simulink model "ex6"  (R2021a)
settings: Solver=VariableStepAuto  StartTime=0.0  StopTime=20  RelTol=1e-8
values from neighbouring files (symbols this model uses):
  gamma = 10    [aae666_hw8_ex6.m]
  theta = 0.5    [aae666_hw8_ex6.m]
settings Model: Creator=Tomo  LastModifiedBy=Tomo

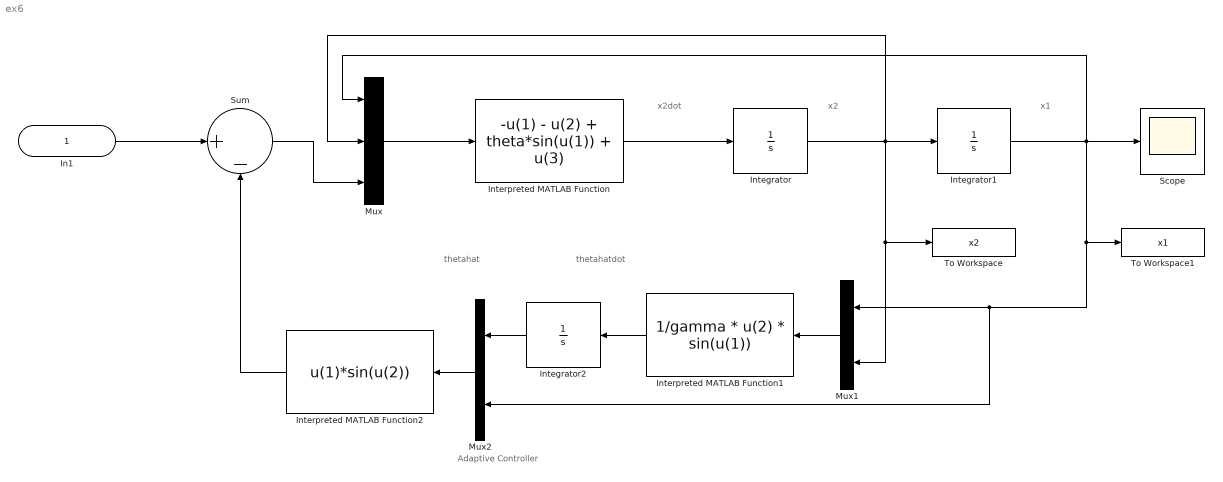
== system ex6 ==
  note: thetahat
  note: Adaptive Controller
  note: x2dot
  note: x2
  note: x1
  note: thetahatdot
  In1 : Inport
  Integrator : Integrator
  Integrator1 : Integrator  InitialCondition=1
  Integrator2 : Integrator
  Interpreted MATLAB Function : MATLABFcn  MATLABFcn=-u(1) - u(2) + theta*sin(u(1)) + u(3)
  Interpreted MATLAB Function1 : MATLABFcn  MATLABFcn=1/gamma * u(2) * sin(u(1))
  Interpreted MATLAB Function2 : MATLABFcn  MATLABFcn=u(1)*sin(u(2))
  Mux : Mux  Inputs=3
  Mux1 : Mux  Inputs=2
  Mux2 : Mux  Inputs=2
  Scope : Scope
  Sum : Sum  Inputs=|+-
  To Workspace : ToWorkspace  VariableName=x2  SaveFormat=Structure With Time  SampleTime=-1
  To Workspace1 : ToWorkspace  VariableName=x1  SaveFormat=Structure With Time  SampleTime=-1
  wires:
  Interpreted MATLAB Function/1 -> Integrator/1
  Integrator/1 -> To Workspace/1, Mux1/2, Integrator1/1, Mux/2
  Integrator1/1 -> To Workspace1/1, Mux2/2, Mux1/1, Mux/1, Scope/1
  In1/1 -> Sum/1
  Sum/1 -> Mux/3
  Mux/1 -> Interpreted MATLAB Function/1
  Mux1/1 -> Interpreted MATLAB Function1/1
  Interpreted MATLAB Function1/1 -> Integrator2/1
  Interpreted MATLAB Function2/1 -> Sum/2
  Integrator2/1 -> Mux2/1
  Mux2/1 -> Interpreted MATLAB Function2/1
